simulink model "remans1"  (R2020a)
settings: Solver=VariableStepAuto  StartTime=0.0  StopTime=3  RelTol=1e-3
libraries: powerlib x23, powerlib_meascontrol x3, simulink x1, eePowerMeasurement x1
settings Model: Creator=Jithinkrishna V M  LastModifiedBy=Jithinkrishna V M

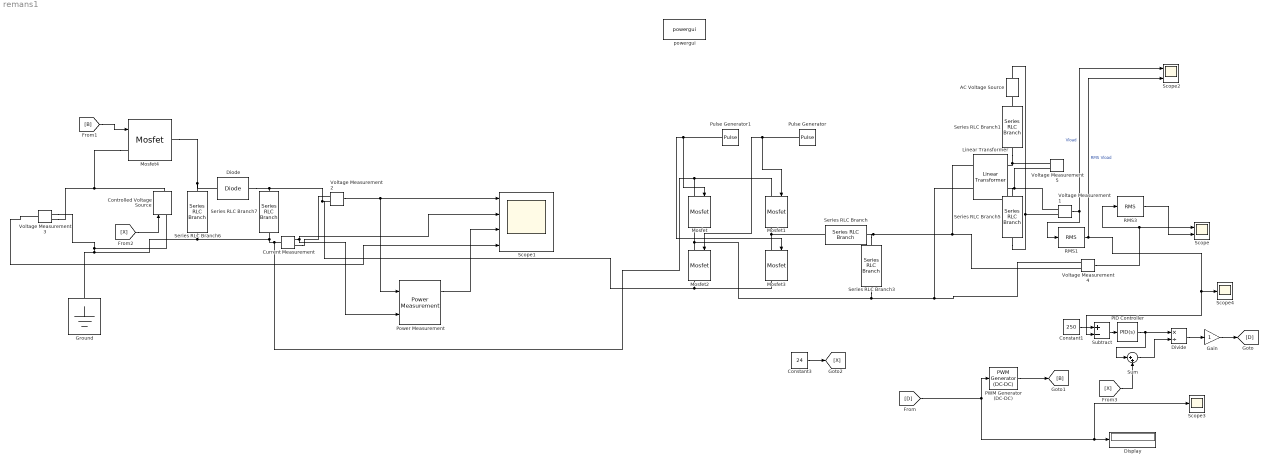
== system remans1 ==
  AC Voltage Source : powerlib/Electrical Sources/AC Voltage Source  Amplitude=352  Phase=0  Frequency=50  SampleTime=0  Measurements=None  BusType=swing  Pref=10e3  Qref=0  Qmin=-inf  Qmax=+inf
  Constant1 : Constant  Value=250
  Constant3 : Constant  Value=24
  Controlled Voltage Source : powerlib/Electrical Sources/Controlled Voltage Source  Initialize=on  Source_Type=DC  Amplitude=0  Phase=0  Frequency=0  Measurements=None
  Current Measurement : powerlib/Measurements/Current Measurement  PhasorSimulation=off  OutputType=Complex  PSBequivalent=0
  Diode : powerlib/Power Electronics/Diode  Ron=0  Lon=0  Vf=0  IC=0  UseSnubber=0  Rs=inf  Cs=250e-9  Measurements=off
  Display : Display
  Divide : Product  Inputs=*/
  Gain : Gain
  Ground : powerlib/Elements/Ground  LConnTagsString=a
  Linear Transformer : powerlib/Elements/Linear Transformer  UNITS=pu  NominalPower=[ 1000 50]  winding1="[ 400  0.002  0.08 ]"  winding2="[ 400  0.002  0.08 ]"  ThreeWindings=off  winding3=[ 315e3 0.002 0.08 ]  RmLm=[ 50 50 ]  Measurements=None  DataType=off
  Mosfet{,1..3} (4 alike) : powerlib/Power Electronics/Mosfet  Ron=0.1  Lon=0  Rd=0.01  Vfd=0  IC=0  Rs=1e5  Cs=inf  Measurements=on
  Mosfet4 : powerlib/Power Electronics/Mosfet  Ron=0.1  Lon=0  Rd=0.01  Vfd=0  IC=0  Rs=inf  Cs=inf  Measurements=off
  PID Controller : simulink/Continuous/PID Controller  Controller=PID  Form=Parallel  TimeDomain=Continuous-time  UseExternalTs=off  SampleTime=-1  IntegratorMethod=Forward Euler  FilterMethod=Forward Euler  ControllerParametersSource=internal  P=.01  I=1  D=.01  UseFilter=on  N=100  TunerSelectOption=Transfer Function Based (PID Tuner App)  InitialConditionSource=internal  InitialConditionForIntegrator=0  InitialConditionForFilter=0  DifferentiatorICPrevScaledInput=0  ExternalReset=none  TrackingMode=off  Kt=1  LimitOutput=off  UpperSaturationLimit=inf  LowerSaturationLimit=-inf  LinearizeAsGain=on  AntiWindupMode=none  Kb=1  POutMin=[]  POutMax=[]  IOutMin=[]  IOutMax=[]  DOutMin=[]  DOutMax=[]  NOutMin=[]  NOutMax=[]  SumOutMin=[]  SumOutMax=[]  SaturationOutMin=[]  SaturationOutMax=[]  PParamMin=[]  PParamMax=[]  IParamMin=[]  IParamMax=[]  DParamMin=[]  DParamMax=[]  NParamMin=[]  NParamMax=[]  KbParamMin=[]  KbParamMax=[]  KtParamMin=[]  KtParamMax=[]  KbOutMin=[]  KbOutMax=[]  KtOutMin=[]  KtOutMax=[]  IntegratorOutMin=[]  IntegratorOutMax=[]  FilterOutMin=[]  FilterOutMax=[]  SumI1OutMin=[]  SumI1OutMax=[]  SumI2OutMin=[]  SumI2OutMax=[]  SumI3OutMin=[]  SumI3OutMax=[]  SumI4OutMin=[]  SumI4OutMax=[]  SumDOutMin=[]  SumDOutMax=[]  DifferentiatorOutMin=[]  DifferentiatorOutMax=[]  FilterDiffOutCoefMin=[]  FilterDiffOutCoefMax=[]  ReciprocalOutMin=[]  ReciprocalOutMax=[]  SumDenOutMin=[]  SumDenOutMax=[]  SumNumOutMin=[]  SumNumOutMax=[]  DivideOutMin=[]  DivideOutMax=[]  UdiffTsProdOutMin=[]  UdiffTsProdOutMax=[]  NTsProdOutMin=[]  NTsProdOutMax=[]  UintegralTsProdOutMin=[]  UintegralTsProdOutMax=[]  UngainTsProdOutMin=[]  UngainTsProdOutMax=[]  IntegratorContinuousStateAttributes=''  IntegratorStateMustResolveToSignalObject=off  IntegratorRTWStateStorageClass=Auto  FilterContinuousStateAttributes=''  FilterStateMustResolveToSignalObject=off  FilterRTWStateStorageClass=Auto  ParallelPVariant=InternalParameters  IdealPVariant=Disabled  IVariant=InternalParameters  DVariant=InternalParameters  IntegratorVariant=Continuous  SatVariant=Disabled  AWVariant=Passthrough  PCopyVariant=Disabled  TRVariant=Disabled  FdbkBlocksVariant=Forward  IdealPFdbkVariant=Disabled  SatFdbkVariant=Disabled  DerivativeFilterVariant=ContFilter  NVariant=InternalParameters  NCopyVariant=Disabled  FilterICVariant=InternalICsFilter  IntegratorICVariant=InternalICs  ExternalResetVariant=Disabled  TRSumVariant=Passthrough  SumFdbkVariant=Disabled  SumVariant=Sum_PID  TsampFilterVariant=InternalTs  TsampNgainVariant=Passthrough  TsampIntegralVariant=Passthrough
  PWM Generator (DC-DC) : powerlib_meascontrol/Pulse & Signal Generators/PWM Generator (DC-DC)  Fsw=20000  Ts=0
  Power Measurement : eePowerMeasurement/Power Measurement  LabelModeActiveChoice=Continuous  F=60  K=[0 1 2 3]  Ts=0
      settings: SourceProductBaseCode=PS
  Pulse Generator : DiscretePulseGenerator  PulseType=Time based  Amplitude=10  Period=.02  PulseWidth=50  PhaseDelay=.01
  Pulse Generator1 : DiscretePulseGenerator  PulseType=Time based  Amplitude=10  Period=.02  PulseWidth=50
  RMS1 : powerlib_meascontrol/Measurements/RMS  TrueRMS=on  Freq=50  RMSInit=0  Ts=0
  RMS3 : powerlib_meascontrol/Measurements/RMS  TrueRMS=on  Freq=50  RMSInit=1  Ts=0
  Scope : Scope  NumInputPorts=2
  Scope1 : Scope  NumInputPorts=4
  Scope2 : Scope  NumInputPorts=2
  Scope3 : Scope
  Scope4 : Scope
  Series RLC Branch : powerlib/Elements/Series RLC Branch  LConnTagsString=__new0  RConnTagsString=__new0  BranchType=L  Resistance=1  Inductance=10e-3  SetiL0=off  InitialCurrent=0  Capacitance=1e-6  Setx0=off  InitialVoltage=0  Measurements=None
  Series RLC Branch1 : powerlib/Elements/Series RLC Branch  LConnTagsString=__new0  RConnTagsString=__new0  BranchType=R  Resistance=2  Inductance=1.5e-3  SetiL0=off  InitialCurrent=0  Capacitance=1e-6  Setx0=off  InitialVoltage=0  Measurements=None
  Series RLC Branch3 : powerlib/Elements/Series RLC Branch  LConnTagsString=__new0  RConnTagsString=__new0  BranchType=C  Resistance=1  Inductance=1e-3  SetiL0=off  InitialCurrent=0  Capacitance=1e-3  Setx0=off  InitialVoltage=0  Measurements=None
  Series RLC Branch5 : powerlib/Elements/Series RLC Branch  LConnTagsString=__new0  RConnTagsString=__new0  BranchType=R  Resistance=98  Inductance=1.5e-3  SetiL0=off  InitialCurrent=0  Capacitance=1e-6  Setx0=off  InitialVoltage=0  Measurements=None
  Series RLC Branch6 : powerlib/Elements/Series RLC Branch  LConnTagsString=__new0  RConnTagsString=__new0  BranchType=L  Resistance=1  Inductance=1.5e-3  SetiL0=off  InitialCurrent=0  Capacitance=1e-6  Setx0=off  InitialVoltage=0  Measurements=None
  Series RLC Branch7 : powerlib/Elements/Series RLC Branch  LConnTagsString=__new0  RConnTagsString=__new0  BranchType=C  Resistance=1  Inductance=1.5e-3  SetiL0=off  InitialCurrent=0  Capacitance=2.2e-3  Setx0=off  InitialVoltage=0  Measurements=None
  Subtract : Sum  Inputs=+-
  Sum : Sum  Inputs=|++
  Voltage Measurement{1..5} (5 alike) : powerlib/Measurements/Voltage Measurement  PhasorSimulation=off  OutputType=Complex  PSBequivalent=0
  powergui : powerlib/powergui  Priority=1  SimulationMode=Continuous  SampleTime=1e-4  frequency=60  Iterations=50  frequencyindice=0  Pbase=100e6  ErrMax=1e-4  UnitsV=kV  UnitsW=MW  buscounter=0  FunctionMessages=off  echomessages=off  EnableUseOfTLC=off  CurrentSourceSwitches=off  DisableSnubberDevices=off  DisableRonSwitches=off  DisableVfSwitches=off  DisplayEquations=off  AutomaticDiscreteSolvers=off  SolverType=Tustin/Backward Euler (TBE)  Interpol=off  ExternalGateDelay=off  methode=off  Ts=100  x0status=blocks  SPID=on  SwTol=0  HookPort=off  NonlinearTolerance=1e-4  nMaxIteration=100  ContinueOnMaxIteration=off  RestoreLinks=warning  ResistiveCurrentMeasurement=off  Frange=[0:2:500]  Ylog=off  Xlog=on  ShowGrid=off  save=off  variable=ZData  structure=0  ZoomFFT=off  StartTime=0.0  cycles=1  DisplayStyle=1  fundamental=60  FreqAxis=off  MaxFrequency=1000  frequencyindicesteady=1  RmsSteady=1  display=off
  wires:
  Pulse Generator1/1 -> Mosfet3/1, Mosfet/1
  Pulse Generator/1 -> Mosfet2/1, Mosfet1/1
  [B] -> Mosfet4/1
  PWM Generator (DC-DC)/1 -> [B]
  Power Measurement/1 -> Scope1/3
  Current Measurement/1 -> Power Measurement/2, Scope1/2
  Voltage Measurement2/1 -> Power Measurement/1, Scope1/1
  Voltage Measurement3/1 -> Scope1/4
  [D] -> PWM Generator (DC-DC)/1, Scope3/1, Display/1
  Voltage Measurement4/1 -> RMS3/1, Scope/1
  RMS3/1 -> Scope/2
  Voltage Measurement1/1 -> Scope2/1, RMS1/1  "Vload"
  RMS1/1 -> Scope4/1, Subtract/2, Scope2/2  "RMS Vload"
  Constant1/1 -> Subtract/1
  [X] -> Sum/2
  Sum/1 -> Divide/2
  Divide/1 -> Gain/1
  Gain/1 -> [D]
  Subtract/1 -> PID Controller/1
  PID Controller/1 -> Sum/1, Divide/1
  Constant3/1 -> [X]
  [X] -> Controlled Voltage Source/1
  connections:
  Series RLC Branch3/LConn1 -- Linear Transformer/LConn1 -- Voltage Measurement4/LConn2 -- Series RLC Branch/RConn1
  Diode/LConn1 -- Series RLC Branch7/LConn1 -- Mosfet3/RConn1 -- Mosfet2/RConn1 -- Voltage Measurement2/LConn2
  Mosfet2/LConn1 -- Voltage Measurement4/LConn1 -- Linear Transformer/LConn2 -- Series RLC Branch3/RConn1 -- Mosfet/RConn1
  Series RLC Branch6/LConn1 -- Diode/RConn1 -- Mosfet4/RConn1
  Mosfet4/LConn1 -- Controlled Voltage Source/RConn1 -- Voltage Measurement3/LConn1
  Series RLC Branch7/RConn1 -- Mosfet1/LConn1 -- Mosfet/LConn1 -- Current Measurement/LConn1 -- Series RLC Branch6/RConn1 -- Controlled Voltage Source/LConn1 -- Voltage Measurement3/LConn2 -- Ground/LConn1
  Current Measurement/RConn1 -- Voltage Measurement2/LConn1
  Mosfet1/RConn1 -- Mosfet3/LConn1 -- Series RLC Branch/LConn1
  Series RLC Branch1/RConn1 -- Linear Transformer/RConn1 -- Voltage Measurement5/LConn1
  Series RLC Branch5/LConn1 -- Voltage Measurement5/LConn2 -- Linear Transformer/RConn2 -- Voltage Measurement1/LConn1
  Series RLC Branch1/LConn1 -- AC Voltage Source/RConn1
  Series RLC Branch5/RConn1 -- AC Voltage Source/LConn1 -- Voltage Measurement1/LConn2
